simulink model "simulation_CP_compacteur"  (R2015b)
settings: Solver=ode23tb  SolverMode=SingleTasking  StartTime=0.0  StopTime=40  FixedStep=1e-3  MaxStep=1e-3
libraries: fl_lib x24, nesl_utility x16, elec_lib x5, sdl_lib x1
settings Model: Creator=rems7881  LastModifiedBy=utilisateur
settings SolverCC: ZeroCrossAlgorithm=Adaptive  AlgebraicLoopSolver=LineSearch
settings DataIOCC: LimitDataPoints=off
settings DebuggingCC: AllowSymbolicDim=on  SFUnexpectedBacktrackingDiag=error  SFNoUnconditionalDefaultTransitionDiag=error
settings ModelReferenceCC: PropagateSignalLabelsOutOfModel=on
settings GRTTargetCC: TargetLangStandard=C99 (ISO)
settings ConfigComp: CovMetricSettings=dwe  CovHtmlReporting=off  CovSaveCumulativeToWorkspaceVar=off  CovSaveSingleToWorkspaceVar=off  CovModelRefEnable=Off  CovExternalEMLEnable=on

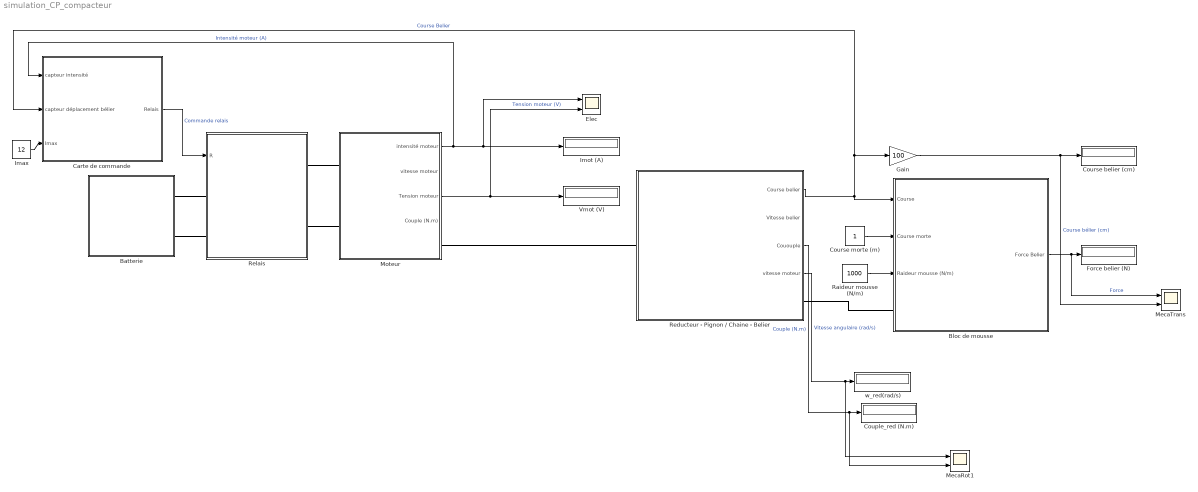
== system simulation_CP_compacteur ==
  Batterie : Subsystem
      mask Display: image('H:\Dropbox\Laurent\IMATEACHER\2020-2021\Enseignements\SI1\Sequences\Sequence2_EnergieSysteme\Ressources\SIMU\TP_SIMU_COMPACTEUR_ELEVES\IMAGES\BBB10.jpg')
  Bloc de mousse : Subsystem
      mask Display: image('H:\Dropbox\Laurent\IMATEACHER\2020-2021\Enseignements\SI1\Sequences\Sequence2_EnergieSysteme\Ressources\SIMU\TP_SIMU_COMPACTEUR_ELEVES\IMAGES\mousse.jpg')
  Carte de commande : Subsystem
      mask Display: image('H:\Dropbox\Laurent\IMATEACHER\2020-2021\Enseignements\SI1\Sequences\Sequence2_EnergieSysteme\Ressources\SIMU\TP_SIMU_COMPACTEUR_ELEVES\IMAGES\carte.png')
  Couple_red (N.m) : Display
  Course belier (cm) : Display
  Course morte (m) : Constant
  Elec : Scope  NumInputPorts=2
  Force belier (N) : Display
  Gain : Gain  Gain=100
  Imax : Constant  Value=12
  Imot (A) : Display
  MecaRot1 : Scope  NumInputPorts=2
  MecaTrans : Scope  NumInputPorts=2
  Moteur : Subsystem  mask{R=0.5, L=0.16e-3, K=0.06, Fv=0.06*(1-0.95)/180, Fs=0.06*(1-0.95), J=0.0006}
      mask prompts: R "Resistance (omhs)"; L "Inductance (H)"; K "Constante vitesse (V/(rad/s))"; Fv "Frottement visqueux (N.m/(rad/s))"; Fs "Frottement sec"; J "Inertie (kg.m²)"
      mask Display: image('H:\Dropbox\Laurent\IMATEACHER\2020-2021\Enseignements\SI1\Sequences\Sequence2_EnergieSysteme\Ressources\SIMU\TP_SIMU_COMPACTEUR_ELEVES\IMAGES\moteur.png')
  Raideur mousse (N/m) : Constant  Value=1000
  Reducteur - Pignon / Chaine - Belier : Subsystem  mask{rend=0.29}
      mask prompts: rend "Rendement global"
      mask Display: image('H:\Dropbox\Laurent\IMATEACHER\2020-2021\Enseignements\SI1\Sequences\Sequence2_EnergieSysteme\Ressources\SIMU\TP_SIMU_COMPACTEUR_ELEVES\IMAGES\reduct_chaine.png')
  Relais : Subsystem
      mask Display: image('H:\Dropbox\Laurent\IMATEACHER\2020-2021\Enseignements\SI1\Sequences\Sequence2_EnergieSysteme\Ressources\SIMU\TP_SIMU_COMPACTEUR_ELEVES\IMAGES\relais.png')
  Vmot (V) : Display
  w_red(rad/s) : Display
  wires:
  Carte de commande/1(Relais) -> Relais/1(R)  "Commande relais"
  Imax/1 -> Carte de commande/3(Imax)
  Moteur/1(intensité moteur) -> Elec/1, Imot (A)/1, Carte de commande/1(capteur intensité)  "Intensité moteur (A)"
  Reducteur - Pignon / Chaine - Belier/1(Course belier) -> Carte de commande/2(capteur déplacement bélier), Gain/1, Bloc de mousse/1(Course)  "Course Belier"
  Bloc de mousse/1(Force Belier) -> MecaTrans/1, Force belier (N)/1  "Force"
  Gain/1 -> MecaTrans/2, Course belier (cm)/1  "Course bélier (cm)"
  Course morte (m)/1 -> Bloc de mousse/2(Course morte)
  Raideur mousse (N/m)/1 -> Bloc de mousse/3(Raideur mousse (N/m))
  Moteur/3(Tension moteur) -> Elec/2, Vmot (V)/1  "Tension moteur (V)"
  Reducteur - Pignon / Chaine - Belier/4(vitesse moteur) -> MecaRot1/1, w_red(rad/s)/1  "Vitesse angulaire (rad/s)"
  Reducteur - Pignon / Chaine - Belier/3(Cououple) -> MecaRot1/2, Couple_red (N.m)/1  "Couple (N.m)"
  connections:
  Moteur/LConn1 -- Relais/RConn1
  Moteur/LConn2 -- Relais/RConn2
  Reducteur - Pignon / Chaine - Belier/LConn1 -- Moteur/RConn1
  Reducteur - Pignon / Chaine - Belier/RConn1 -- Bloc de mousse/LConn1
  Batterie/RConn1 -- Relais/LConn1
  Batterie/RConn2 -- Relais/LConn2

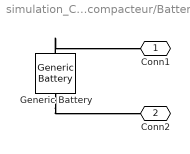
== system simulation_CP_compacteur/Batterie ==
  Generic Battery : elec_lib/Sources/Generic Battery  Vnom=12 V  R1=0.5 Ohm  prm_AH=1  AH=50 hr*A  AH0=50 hr*A  V1=11.5 V  AH1=25 hr*A  prm_R2=1  R2=2e+3 Ohm
  Conn1 : PMIOPort  Port=1  Side=Right
  Conn2 : PMIOPort  Port=2  Side=Right
  connections:
  Generic Battery/LConn1 -- Conn1/RConn1
  Generic Battery/RConn1 -- Conn2/RConn1

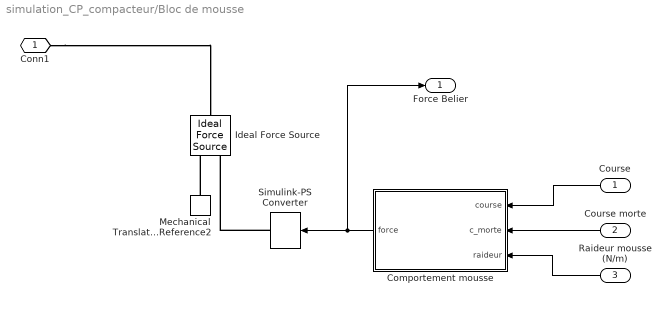
== system simulation_CP_compacteur/Bloc de mousse ==
  Course : Inport
  Course morte : Inport  Port=2
  Raideur mousse (N/m) : Inport  Port=3
  Comportement mousse : MATLAB Function  TreatAsAtomicUnit=on
  Ideal Force Source : fl_lib/Mechanical/Mechanical Sources/Ideal Force Source
  Mechanical Translational Reference2 : fl_lib/Mechanical/Translational Elements/Mechanical Translational Reference
  Simulink-PS Converter : nesl_utility/Simulink-PS Converter  PhysicalDomain=network_engine_domain  SubClassName=ps_input  LeftPortType=input  RightPortType=output  PseudoPeriodic=off  Frequencies=[]  NoiseDistribution=none  NoiseParameters=[]  Unit=N  AffineConversion=off  InputFiltering=on  SimscapeFilterOrder=1  InputFilterTimeConstant=.001  UdotUserProvided=1
  Conn1 : PMIOPort  Port=1  Side=Left
  Force Belier : Outport
  wires:
  Comportement mousse/1(force) -> Force Belier/1, Simulink-PS Converter/1
  Course/1 -> Comportement mousse/1(course)
  Course morte/1 -> Comportement mousse/2(c_morte)
  Raideur mousse (N/m)/1 -> Comportement mousse/3(raideur)
  connections:
  Mechanical Translational Reference2/LConn1 -- Ideal Force Source/RConn2
  Simulink-PS Converter/RConn1 -- Ideal Force Source/RConn1
  Conn1/RConn1 -- Ideal Force Source/LConn1

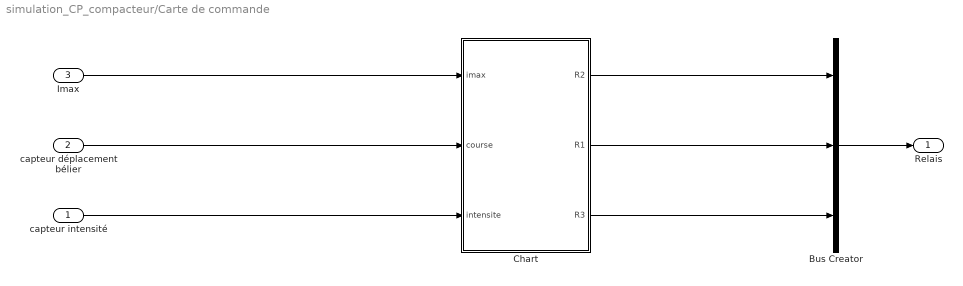
== system simulation_CP_compacteur/Carte de commande ==
  capteur intensité : Inport
  capteur déplacement bélier : Inport  Port=2
  Imax : Inport  Port=3
  Bus Creator : BusCreator  Inputs=3
  Chart : Stateflow chart  TreatAsAtomicUnit=on
  Relais : Outport
  wires:
  capteur intensité/1 -> Chart/3(intensite)
  Chart/1(R2) -> Bus Creator/1
  Imax/1 -> Chart/1(imax)
  capteur déplacement bélier/1 -> Chart/2(course)
  Chart/2(R1) -> Bus Creator/2
  Chart/3(R3) -> Bus Creator/3
  Bus Creator/1 -> Relais/1

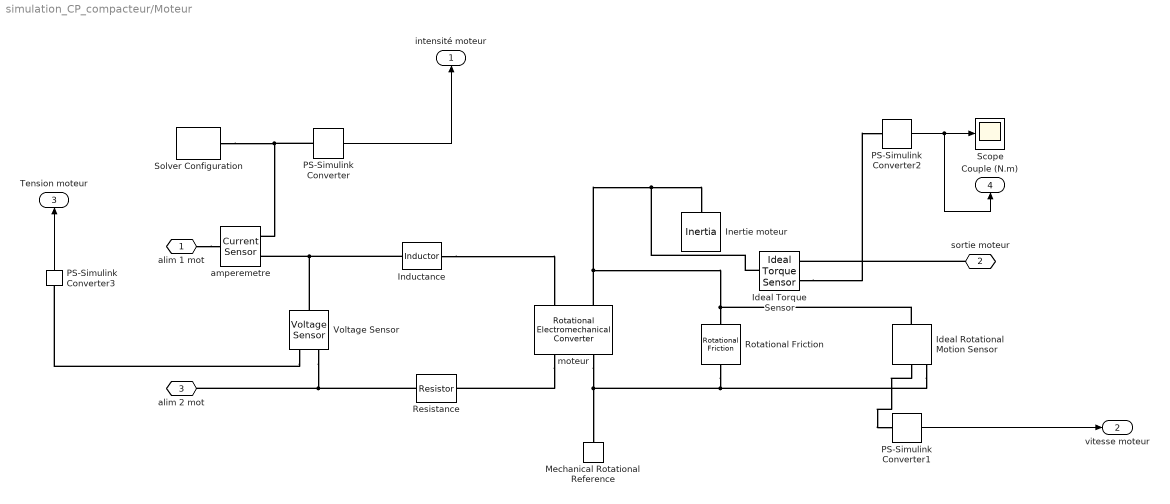
== system simulation_CP_compacteur/Moteur ==
  Ideal Rotational Motion Sensor : fl_lib/Mechanical/Mechanical Sensors/Ideal Rotational Motion Sensor  offset=0 rad
  Ideal Torque Sensor : fl_lib/Mechanical/Mechanical Sensors/Ideal Torque Sensor
  Inductance : fl_lib/Electrical/Electrical Elements/Inductor  l=L H  r=0 Ohm  g=1e-9 1/Ohm  i_specify=off  i_priority=High  i=0 A  v_specify=off  v_priority=High  v=0 V  i_L_specify=on  i_L_priority=High  i_L=0 A
  Inertie moteur : fl_lib/Mechanical/Rotational Elements/Inertia  inertia=J kg*m^2  w_specify=on  w_priority=High  w=0 rad/s  t_specify=off  t_priority=High  t=0 N*m
  Mechanical Rotational Reference : fl_lib/Mechanical/Rotational Elements/Mechanical Rotational Reference
  PS-Simulink Converter : nesl_utility/PS-Simulink Converter  PhysicalDomain=network_engine_domain  SubClassName=ps_output  LeftPortType=input  RightPortType=output  PseudoPeriodic=off  Frequencies=[]  Unit=A  AffineConversion=off
  PS-Simulink Converter1 : nesl_utility/PS-Simulink Converter  PhysicalDomain=network_engine_domain  SubClassName=ps_output  LeftPortType=input  RightPortType=output  PseudoPeriodic=off  Frequencies=[]  Unit=rad/s  AffineConversion=off
  PS-Simulink Converter2 : nesl_utility/PS-Simulink Converter  PhysicalDomain=network_engine_domain  SubClassName=ps_output  LeftPortType=input  RightPortType=output  PseudoPeriodic=off  Frequencies=[]  Unit=N*m  AffineConversion=off
  PS-Simulink Converter3 : nesl_utility/PS-Simulink Converter  PhysicalDomain=network_engine_domain  SubClassName=ps_output  LeftPortType=input  RightPortType=output  PseudoPeriodic=off  Frequencies=[]  Unit=V  AffineConversion=off
  Resistance : fl_lib/Electrical/Electrical Elements/Resistor  R=R Ohm  i_specify=off  i_priority=High  i=0 A  v_specify=off  v_priority=High  v=0 V
  Rotational Friction : fl_lib/Mechanical/Rotational Elements/Rotational Friction  brkwy_trq=Fs N*m  Col_trq=Fs N*m  visc_coef=Fv N*m/(rad/s)  trans_coef=10 s/rad  vel_thr=1e-4 rad/s  w_specify=off  w_priority=High  w=0 rad/s  t_specify=off  t_priority=High  t=0 N*m
  Scope : Scope
  Solver Configuration : nesl_utility/Solver Configuration  PhysicalDomain=network_engine_domain  SubClassName=solver  LeftPortType=input  RightPortType=generic  Accelerate=off  Tones=[]  Harmonics=[]  SimulateNoise=off  Profile=off  UseLocalSampling=off  EnableSwitchedLinearOptims=on  FrequencyDomain=off  UseCCode=off  RelTol=0.001  AbsTol=1e-06  MinStep=1e-09  ToWorkspace=off  RevertToSquareIcSolve=off  NumHomotopyIterations=100  PhasorMode=off  PhasorModeNumHarmonics=1  DoDC=off  ResidualTolerance=1e-9  UseLocalSolver=off  LocalSolverChoice=NE_BACKWARD_EULER_ADVANCER  LocalSolverSampleTime=.001  DoFixedCost=off  MaxNonlinIter=3  MaxModeIter=2  LinearAlgebra=Sparse  DelaysMemoryBudget=1024  AutomaticFiltering=on  FilteringTimeConstant=0.001
  Voltage Sensor : fl_lib/Electrical/Electrical Sensors/Voltage Sensor
  amperemetre : fl_lib/Electrical/Electrical Sensors/Current Sensor
  moteur : fl_lib/Electrical/Electrical Elements/Rotational Electromechanical Converter  K=K V/(rad/s)  i_specify=off  i_priority=High  i=0 A  v_specify=off  v_priority=High  v=0 V  t_specify=off  t_priority=High  t=0 N*m  w_specify=off  w_priority=High  w=0 rad/s
  alim 1 mot : PMIOPort  Port=1  Side=Left
  sortie moteur : PMIOPort  Port=2  Side=Right
  alim 2 mot : PMIOPort  Port=3  Side=Left
  intensité moteur : Outport
  vitesse moteur : Outport  Port=2
  Tension moteur : Outport  Port=3
  Couple (N.m) : Outport  Port=4
  wires:
  PS-Simulink Converter1/1 -> vitesse moteur/1
  PS-Simulink Converter/1 -> intensité moteur/1
  PS-Simulink Converter2/1 -> Couple (N.m)/1, Scope/1
  PS-Simulink Converter3/1 -> Tension moteur/1
  connections:
  sortie moteur/RConn1 -- Ideal Torque Sensor/RConn1
  Ideal Rotational Motion Sensor/RConn1 -- Mechanical Rotational Reference/LConn1 -- moteur/RConn2 -- Rotational Friction/RConn1
  Ideal Rotational Motion Sensor/RConn2 -- PS-Simulink Converter1/LConn1
  Inductance/LConn1 -- Voltage Sensor/LConn1 -- amperemetre/RConn2
  Inductance/RConn1 -- moteur/LConn1
  PS-Simulink Converter/LConn1 -- Solver Configuration/RConn1 -- amperemetre/RConn1
  Resistance/LConn1 -- Voltage Sensor/RConn2 -- alim 2 mot/RConn1
  moteur/RConn1 -- Resistance/RConn1
  alim 1 mot/RConn1 -- amperemetre/LConn1
  Ideal Rotational Motion Sensor/LConn1 -- Rotational Friction/LConn1 -- moteur/LConn2 -- Ideal Torque Sensor/LConn1 -- Inertie moteur/LConn1
  Ideal Torque Sensor/RConn2 -- PS-Simulink Converter2/LConn1
  Voltage Sensor/RConn1 -- PS-Simulink Converter3/LConn1

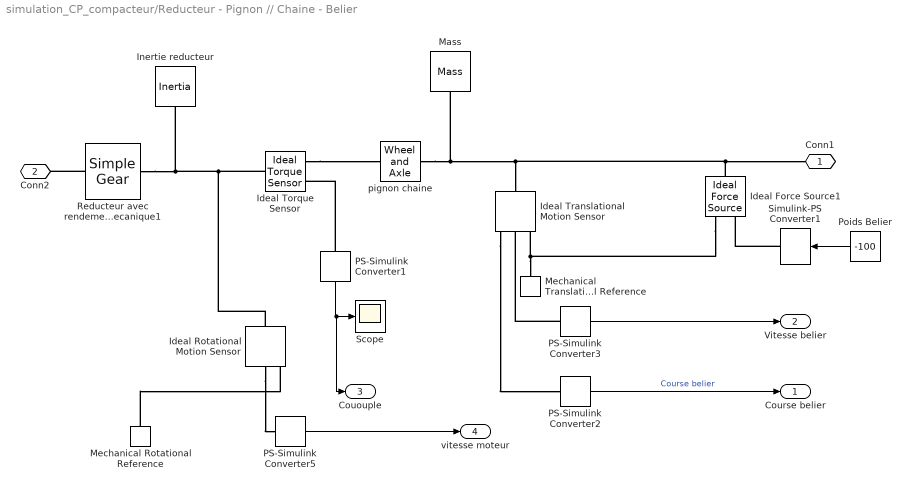
== system simulation_CP_compacteur/Reducteur - Pignon // Chaine - Belier ==
  Ideal Force Source1 : fl_lib/Mechanical/Mechanical Sources/Ideal Force Source
  Ideal Rotational Motion Sensor : fl_lib/Mechanical/Mechanical Sensors/Ideal Rotational Motion Sensor  offset=0 rad
  Ideal Torque Sensor : fl_lib/Mechanical/Mechanical Sensors/Ideal Torque Sensor
  Ideal Translational Motion Sensor : fl_lib/Mechanical/Mechanical Sensors/Ideal Translational Motion Sensor  offset=0 m
  Inertie reducteur : fl_lib/Mechanical/Rotational Elements/Inertia  inertia=1e-5 kg*m^2  w_specify=on  w_priority=High  w=0 rad/s  t_specify=off  t_priority=High  t=0 N*m
  Mass : fl_lib/Mechanical/Translational Elements/Mass  mass=10 kg  v_specify=on  v_priority=High  v=0 m/s  f_specify=off  f_priority=High  f=0 N
  Mechanical Rotational Reference : fl_lib/Mechanical/Rotational Elements/Mechanical Rotational Reference
  Mechanical Translational Reference : fl_lib/Mechanical/Translational Elements/Mechanical Translational Reference
  PS-Simulink Converter1 : nesl_utility/PS-Simulink Converter  PhysicalDomain=network_engine_domain  SubClassName=ps_output  LeftPortType=input  RightPortType=output  PseudoPeriodic=off  Frequencies=[]  Unit=N*m  AffineConversion=off
  PS-Simulink Converter2 : nesl_utility/PS-Simulink Converter  PhysicalDomain=network_engine_domain  SubClassName=ps_output  LeftPortType=input  RightPortType=output  PseudoPeriodic=off  Frequencies=[]  Unit=1  AffineConversion=off
  PS-Simulink Converter3 : nesl_utility/PS-Simulink Converter  PhysicalDomain=network_engine_domain  SubClassName=ps_output  LeftPortType=input  RightPortType=output  PseudoPeriodic=off  Frequencies=[]  Unit=1  AffineConversion=off
  PS-Simulink Converter5 : nesl_utility/PS-Simulink Converter  PhysicalDomain=network_engine_domain  SubClassName=ps_output  LeftPortType=input  RightPortType=output  PseudoPeriodic=off  Frequencies=[]  Unit=rad/s  AffineConversion=off
  Poids Belier : Constant  Value=-100
  Reducteur avec rendement global de la chaine mecanique1 : sdl_lib/Gears/Simple Gear  ratio=216  rotation_direction=2  friction_model=1  T_noload=0.1 N*m  T_nom=5 N*m  efficiency_nom=0.8  efficiency=rend  mu_visc=[0, 0] N*m/(rad/s)  w_thr=0.01 rad/s  temperature_TLU=[280, 300, 320] K  load_TLU=[1, 5, 10] N*m  efficiency_TLU=[.95, .9, .85]  efficiency_TLU2=[.85, .8, .75; .95, .9, .85; .85, .8, .7]  thermal_mass=50 J/K  T_init=300 K
  Scope : Scope
  Simulink-PS Converter1 : nesl_utility/Simulink-PS Converter  PhysicalDomain=network_engine_domain  SubClassName=ps_input  LeftPortType=input  RightPortType=output  PseudoPeriodic=off  Frequencies=[]  NoiseDistribution=none  NoiseParameters=[]  Unit=N  AffineConversion=off  InputFiltering=off  SimscapeFilterOrder=1  InputFilterTimeConstant=.001  UdotUserProvided=0
  pignon chaine : fl_lib/Mechanical/Mechanisms/Wheel and Axle  R=73.1e-3/2 m  or=1  orient=1  t_specify=off  t_priority=High  t=0 N*m  f_specify=off  f_priority=High  f=0 N
  Conn1 : PMIOPort  Port=1  Side=Right
  Conn2 : PMIOPort  Port=2  Side=Left
  Course belier : Outport
  Vitesse belier : Outport  Port=2
  Cououple : Outport  Port=3
  vitesse moteur : Outport  Port=4
  wires:
  Poids Belier/1 -> Simulink-PS Converter1/1
  PS-Simulink Converter2/1 -> Course belier/1  "Course belier"
  PS-Simulink Converter1/1 -> Cououple/1, Scope/1
  PS-Simulink Converter3/1 -> Vitesse belier/1
  PS-Simulink Converter5/1 -> vitesse moteur/1
  connections:
  Inertie reducteur/LConn1 -- Ideal Rotational Motion Sensor/LConn1 -- Ideal Torque Sensor/LConn1 -- Reducteur avec rendement global de la chaine mecanique1/RConn1
  Reducteur avec rendement global de la chaine mecanique1/LConn1 -- Conn2/RConn1
  Mechanical Translational Reference/LConn1 -- Ideal Force Source1/RConn2 -- Ideal Translational Motion Sensor/RConn1
  PS-Simulink Converter1/LConn1 -- Ideal Torque Sensor/RConn2
  Ideal Torque Sensor/RConn1 -- pignon chaine/LConn1
  Simulink-PS Converter1/RConn1 -- Ideal Force Source1/RConn1
  Ideal Translational Motion Sensor/RConn3 -- PS-Simulink Converter2/LConn1
  Ideal Force Source1/LConn1 -- Conn1/RConn1 -- Mass/LConn1 -- pignon chaine/RConn1 -- Ideal Translational Motion Sensor/LConn1
  PS-Simulink Converter3/LConn1 -- Ideal Translational Motion Sensor/RConn2
  Ideal Rotational Motion Sensor/RConn2 -- PS-Simulink Converter5/LConn1
  Mechanical Rotational Reference/LConn1 -- Ideal Rotational Motion Sensor/RConn1

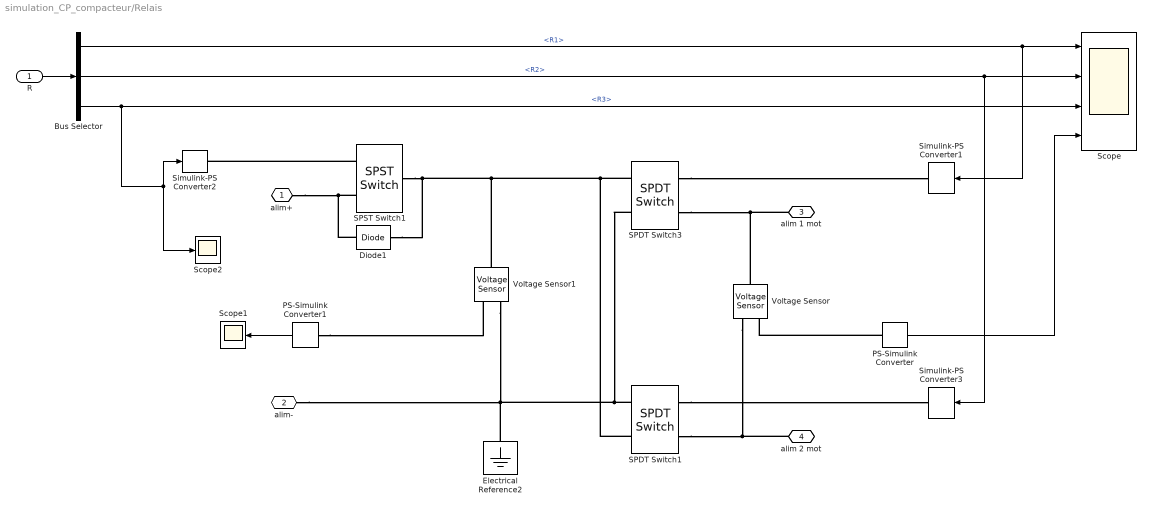
== system simulation_CP_compacteur/Relais ==
  R : Inport
  Bus Selector : BusSelector  OutputSignals=R1,R2,R3
  Diode1 : elec_lib/Semiconductor Devices/Diode  ModelType=1  Vf=0.8 V  Ron=0.001 Ohm  Goff=1e-5 S  Rz=0.3 Ohm  Vz=50 V  C_PWL=0 pF  prmExp=1  I12=[ 0.0137 0.545 ] A  V12=[ 0.6 0.7 ] V  I1=0.0137 A  V1=0.6 V  RS=0.01 Ohm  IS=1e-12 A  Tmeas=25 C  ec=1  BV=Inf V  C_param=1  CJ0=5 pF  VJ=1 V  Mgrad=0.5  Vvec=[ 0.1 10 100 ] V  Cvec=[ 3.5 1 0.4 ] pF  FC=0.5  Q_param=1  Irrm=-7.15 A  iF=4 A  didt=-750 A/us  trr=115 ns  TT=50 ns  tau=100 ns  T_param=1  IS_T2=1.25e-7 A  I1_T2=0.245 A  V1_T2=0.5 V  Tmeas2=125 C  EG_param=1  EG=1.11 eV  XTI_param=1  XTI=3  dBVdT=0 V/K  Tdevice=25 C  Rth=[ 0 10 ] K/W  thermal_mass_parameterization=1  thermal_mass=[ 0 1 ] J/K  thermal_time_constant=[ 0 10 ] s  thermal_mass_initial_temperatures=[ 25 25 ] C
  Electrical Reference2 : fl_lib/Electrical/Electrical Elements/Electrical Reference
  PS-Simulink Converter : nesl_utility/PS-Simulink Converter  PhysicalDomain=network_engine_domain  SubClassName=ps_output  LeftPortType=input  RightPortType=output  PseudoPeriodic=off  Frequencies=[]  Unit=V  AffineConversion=off
  PS-Simulink Converter1 : nesl_utility/PS-Simulink Converter  PhysicalDomain=network_engine_domain  SubClassName=ps_output  LeftPortType=input  RightPortType=output  PseudoPeriodic=off  Frequencies=[]  Unit=1  AffineConversion=off
  SPDT Switch1 : elec_lib/Passive Devices/Switches/SPDT Switch  R_closed=0.01 Ohm  G_open=1e-6 S  Threshold=0 V  Width=0.1 V  model_dynamics=0  t_on=0.001 s  t_off=0.001 s  initial_vT=0 V
  SPDT Switch3 : elec_lib/Passive Devices/Switches/SPDT Switch  R_closed=0.01 Ohm  G_open=1e-6 S  Threshold=0 V  Width=0.1 V  model_dynamics=0  t_on=0.001 s  t_off=0.001 s  initial_vT=0 V
  SPST Switch1 : elec_lib/Passive Devices/Switches/SPST Switch  R_closed=0.01 Ohm  G_open=1e-6 S  Threshold=0 V  Width=0.1 V  model_dynamics=0  t_on=0.001 s  t_off=0.001 s  initial_vT=0 V
  Scope : Scope  NumInputPorts=4
  Scope1 : Scope
  Scope2 : Scope
  Simulink-PS Converter1 : nesl_utility/Simulink-PS Converter  PhysicalDomain=network_engine_domain  SubClassName=ps_input  LeftPortType=input  RightPortType=output  PseudoPeriodic=off  Frequencies=[]  NoiseDistribution=none  NoiseParameters=[]  Unit=V  AffineConversion=off  InputFiltering=off  SimscapeFilterOrder=1  InputFilterTimeConstant=.001  UdotUserProvided=0
  Simulink-PS Converter2 : nesl_utility/Simulink-PS Converter  PhysicalDomain=network_engine_domain  SubClassName=ps_input  LeftPortType=input  RightPortType=output  PseudoPeriodic=off  Frequencies=[]  NoiseDistribution=none  NoiseParameters=[]  Unit=1  AffineConversion=off  InputFiltering=off  SimscapeFilterOrder=1  InputFilterTimeConstant=.001  UdotUserProvided=0
  Simulink-PS Converter3 : nesl_utility/Simulink-PS Converter  PhysicalDomain=network_engine_domain  SubClassName=ps_input  LeftPortType=input  RightPortType=output  PseudoPeriodic=off  Frequencies=[]  NoiseDistribution=none  NoiseParameters=[]  Unit=V  AffineConversion=off  InputFiltering=off  SimscapeFilterOrder=1  InputFilterTimeConstant=.001  UdotUserProvided=0
  Voltage Sensor : fl_lib/Electrical/Electrical Sensors/Voltage Sensor
  Voltage Sensor1 : fl_lib/Electrical/Electrical Sensors/Voltage Sensor
  alim+ : PMIOPort  Port=1  Side=Left
  alim- : PMIOPort  Port=2  Side=Left
  alim 1 mot : PMIOPort  Port=3  Side=Right
  "alim 2 mot " : PMIOPort  Port=4  Side=Right
  wires:
  Bus Selector/3 -> Scope2/1, Simulink-PS Converter2/1, Scope/3  "<R3>"
  Bus Selector/1 -> Simulink-PS Converter1/1, Scope/1  "<R1>"
  Bus Selector/2 -> Simulink-PS Converter3/1, Scope/2  "<R2>"
  R/1 -> Bus Selector/1
  PS-Simulink Converter/1 -> Scope/4
  PS-Simulink Converter1/1 -> Scope1/1
  connections:
  alim+/RConn1 -- SPST Switch1/LConn2 -- Diode1/RConn1
  alim 1 mot/RConn1 -- SPDT Switch3/LConn2 -- Voltage Sensor/LConn1
  "alim 2 mot "/RConn1 -- SPDT Switch1/LConn2 -- Voltage Sensor/RConn2
  SPDT Switch1/LConn1 -- Simulink-PS Converter3/RConn1
  SPDT Switch3/LConn1 -- Simulink-PS Converter1/RConn1
  PS-Simulink Converter/LConn1 -- Voltage Sensor/RConn1
  Voltage Sensor1/RConn2 -- SPDT Switch1/RConn1 -- SPDT Switch3/RConn2 -- Electrical Reference2/LConn1 -- alim-/RConn1
  PS-Simulink Converter1/LConn1 -- Voltage Sensor1/RConn1
  SPST Switch1/LConn1 -- Simulink-PS Converter2/RConn1
  Voltage Sensor1/LConn1 -- SPDT Switch1/RConn2 -- SPDT Switch3/RConn1 -- SPST Switch1/RConn1 -- Diode1/LConn1

== matlab function simulation_CP_compacteur/Bloc de mousse/Comportement mousse ==
  data: course input; force output; c_morte input; raideur input
function force = fcn(course, c_morte, raideur)

if course <= -c_morte % -c_morte = début du compactage
    force = -raideur * (course + c_morte);
else
    force = 0;
end

== stateflow chart simulation_CP_compacteur/Carte de commande/Chart ==
  settings: stateMachineType=MOORE_MACHINE
  state Off
    R1 = 0;
    R2 = 0;
    R3 = 0;
  state Descente
    R1 = 0;
    R2 = 0;
    R3 = 1;
  state Montee
    R1 = 1;
    R2 = 1;
    R3 = 1;
  state stop
    R1 = 0;
    R2 = 0;
    R3 = 0;
  (default) -> Off
  Off -> Descente : after(1,sec)
  Descente -> Montee : [after(0.2,sec) && intensite >= imax]
  Montee -> stop : [course >= 0]
  data: R2 output; R1 output; R3 output; imax input; course input; intensite input
